simulink model "OneDOF"  (R2014b)
settings: Solver=FixedStepAuto  StartTime=0.0  StopTime=10.0  FixedStep=0.01  RelTol=1e-3
values from neighbouring files (symbols this model uses):
  G_dis = (2*zeta*omega_n*s+omega_n^2)/(s^2 + 2*zeta*omega_n*s+omega_n^2)    [OneDOF_mat.m]    (also in damped_passive_system.m)
  G_PD = k_p/(m_p*s^2+dd*s+dp+k_p)    [OneDOF_mat.m]
  G_PID = s*k_p/(m_p*s^3+hd*s^2+(k_p+hp)*s+hi)    [OneDOF_mat.m]
  k_p = 6.32    [OneDOF_mat.m]    (also in TwoDOF_mat.m; damped_passive_system.m)
  m_p = 0.16    [OneDOF_mat.m]    (also in TwoDOF_mat.m; damped_passive_system.m)
  use_step = 0    [OneDOF_mat.m]    (also in TwoDOF_mat.m = 1; damped_passive_system.m)
settings Model: Creator=signat  LastModifiedBy=eric
settings DataIOCC: LimitDataPoints=off  SaveFormat=Dataset
settings OptimizationCC: UseDivisionForNetSlopeComputation=off  LifeSpan=auto  SimCompilerOptimization=off
settings DebuggingCC: SolverPrmCheckMsg=none  FcnCallInpInsideContextMsg=error  FrameProcessingCompatibilityMsg=error  SFUnexpectedBacktrackingDiag=error  SFNoUnconditionalDefaultTransitionDiag=error
settings HardwareCC: ProdBitPerPointer=64  ProdLargestAtomicFloat=Float  ProdIntDivRoundTo=Zero  ProdEndianess=LittleEndian  ProdWordSize=64  ProdHWDeviceType=Intel->x86-64 (Windows64)
settings ModelReferenceCC: PropagateSignalLabelsOutOfModel=on
settings RTWCC: RTWCompilerOptimization=off
settings GRTTargetCC: TargetLangStandard=C99 (ISO)  GeneratePreprocessorConditionals=Use local settings

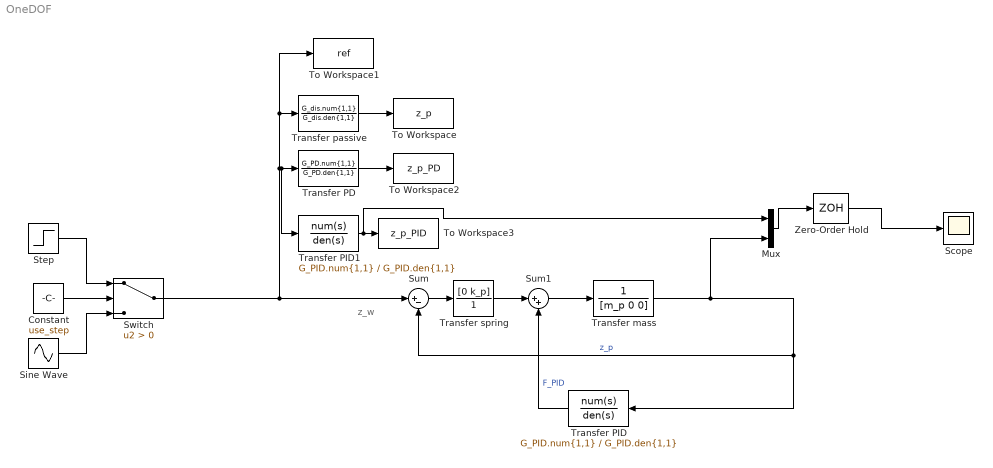
== system OneDOF ==
  note: z_w
  Constant : Constant  Value=use_step
  Mux : Mux  Inputs=2
  Scope : Scope
  Sine Wave : Sin  Amplitude=0.05  SampleTime=0
  Step : Step  After=0.05  SampleTime=0
  Sum : Sum  Inputs=|+-
  Sum1 : Sum  Inputs=|++
  Switch : Switch  Criteria=u2 > Threshold
  To Workspace : ToWorkspace  VariableName=z_p  SaveFormat=Timeseries  SampleTime=-1
  To Workspace1 : ToWorkspace  VariableName=ref  SaveFormat=Timeseries  SampleTime=-1
  To Workspace2 : ToWorkspace  VariableName=z_p_PD  SaveFormat=Timeseries  SampleTime=-1
  To Workspace3 : ToWorkspace  VariableName=z_p_PID  SaveFormat=Timeseries  SampleTime=-1
  Transfer PD : TransferFcn  Numerator=G_PD.num{1,1}  Denominator=G_PD.den{1,1}
  Transfer PID : TransferFcn  Numerator=G_PID.num{1,1}  Denominator=G_PID.den{1,1}
  Transfer PID1 : TransferFcn  Numerator=G_PID.num{1,1}  Denominator=G_PID.den{1,1}
  Transfer mass : TransferFcn  Numerator=1  Denominator=[m_p 0 0]
  Transfer passive : TransferFcn  Numerator=G_dis.num{1,1}  Denominator=G_dis.den{1,1}
  Transfer spring : TransferFcn  Numerator=[0 k_p]  Denominator=1
  Zero-Order Hold : ZeroOrderHold  SampleTime=0.01
  wires:
  Step/1 -> Switch/1
  Sine Wave/1 -> Switch/3
  Constant/1 -> Switch/2
  Transfer passive/1 -> To Workspace/1
  Transfer PD/1 -> To Workspace2/1
  Transfer PID1/1 -> Mux/1, To Workspace3/1
  Sum/1 -> Transfer spring/1
  Switch/1 -> Sum/1, To Workspace1/1, Transfer passive/1, Transfer PID1/1, Transfer PD/1
  Transfer mass/1 -> Mux/2, Transfer PID/1, Sum/2  "z_p"
  Transfer spring/1 -> Sum1/1
  Sum1/1 -> Transfer mass/1
  Transfer PID/1 -> Sum1/2  "F_PID"
  Mux/1 -> Zero-Order Hold/1
  Zero-Order Hold/1 -> Scope/1
